simulink model "neurogrip_adaptive_mpc_closed_loop"  (R2026a)
settings: Solver=FixedStepDiscrete  StopTime=0.4  FixedStep=0.02
model workspace (MAT data in the model file):
  adaptiveMpc = mpc
  adaptiveMpc.Ts = 0.02
  adaptiveMpc.PredictionHorizon = 30
  adaptiveMpc.ControlHorizon = 30
  adaptiveMpc.Model.Plant = ss
  adaptiveMpc.Model.Plant.InputName_ = ["steering_angle_rad"; "d_kappa_rad_s"]
  adaptiveMpc.Model.Plant.InputGroup_.Manipulated = 1
  adaptiveMpc.Model.Plant.InputGroup_.Measured = 2
  adaptiveMpc.Model.Plant.OutputName_ = ["e_y_m"; "e_psi_rad"; "v_y_mps"; "yaw_rate_rps"]
  adaptiveMpc.Model.Plant.OutputGroup_.Measured = [1 2 3 4]
  adaptiveMpc.Model.Plant.IOSize_ = [4 2]
  adaptiveMpc.Model.Plant.Data_ = ltipack.ssdata
  adaptiveMpc.Model.Plant.Data_.a = [1  0.09  0.02  0; 0  1  0  0.02; 0  0  0.463654239616  -0.0414393740331; 0  0  0  0.457235651577]
  adaptiveMpc.Model.Plant.Data_.c = [1  0  0  0; 0  1  0  0; 0  0  1  0; 0  0  0  1]
  adaptiveMpc.Model.Plant.Data_.dx0 = [0; 0; 0; 0]
  adaptiveMpc.Model.Plant.Data_.x0 = [0; 0; 0; 0]
  adaptiveMpc.Model.Plant.Data_.b = [0  0; 0  -0.02; 1.14394485122  0; 1.59636573066  0]
  adaptiveMpc.Model.Plant.Data_.d = [0  0; 0  0; 0  0; 0  0]
  adaptiveMpc.Model.Plant.Data_.u0 = [0; 0]
  adaptiveMpc.Model.Plant.Data_.y0 = [0; 0; 0; 0]
  adaptiveMpc.Model.Plant.Data_.Delay.Input = [0; 0]
  adaptiveMpc.Model.Plant.Data_.Delay.Output = [0; 0; 0; 0]
  adaptiveMpc.Model.Plant.Data_.Delay.Internal = []
  adaptiveMpc.Model.Plant.Data_.Ts = 0.02
  adaptiveMpc.Model.Disturbance = []
  adaptiveMpc.Model.Noise = []
  adaptiveMpc.Model.Nominal.X = [0; 0; 0; 0]
  adaptiveMpc.Model.Nominal.DX = [0; 0; 0; 0]
  adaptiveMpc.Model.Nominal.U = [0; 0]
  adaptiveMpc.Model.Nominal.Y = [0; 0; 0; 0]
  adaptiveMpc.ManipulatedVariables.Min = -0.37
  adaptiveMpc.ManipulatedVariables.Max = 0.37
  adaptiveMpc.ManipulatedVariables.MinECR = 0
  adaptiveMpc.ManipulatedVariables.MaxECR = 0
  adaptiveMpc.ManipulatedVariables.RateMin = -0.05
  adaptiveMpc.ManipulatedVariables.RateMax = 0.05
  adaptiveMpc.ManipulatedVariables.RateMinECR = 0
  adaptiveMpc.ManipulatedVariables.RateMaxECR = 0
  adaptiveMpc.ManipulatedVariables.Target = 'nominal'
  adaptiveMpc.ManipulatedVariables.Name = 'steering_angle_rad'
  adaptiveMpc.ManipulatedVariables.Units = ''
  adaptiveMpc.ManipulatedVariables.ScaleFactor = 1
  adaptiveMpc.ManipulatedVariables.Type = 'continuous'
  adaptiveMpc.OutputVariables(1).Min = -1.5
  adaptiveMpc.OutputVariables(1).Max = 1.5
  adaptiveMpc.OutputVariables(1).MinECR = 1
  adaptiveMpc.OutputVariables(1).MaxECR = 1
  adaptiveMpc.OutputVariables(1).Name = 'e_y_m'
  adaptiveMpc.OutputVariables(1).Units = ''
  adaptiveMpc.OutputVariables(1).ScaleFactor = 1
  adaptiveMpc.OutputVariables(2).Min = -Inf
  adaptiveMpc.OutputVariables(2).Max = Inf
  adaptiveMpc.OutputVariables(2).MinECR = 1
  adaptiveMpc.OutputVariables(2).MaxECR = 1
  adaptiveMpc.OutputVariables(2).Name = 'e_psi_rad'
  adaptiveMpc.OutputVariables(2).Units = ''
  adaptiveMpc.OutputVariables(2).ScaleFactor = 1
  adaptiveMpc.OutputVariables(3).Min = -Inf
  adaptiveMpc.OutputVariables(3).Max = Inf
  adaptiveMpc.OutputVariables(3).MinECR = 1
  adaptiveMpc.OutputVariables(3).MaxECR = 1
  adaptiveMpc.OutputVariables(3).Name = 'v_y_mps'
  adaptiveMpc.OutputVariables(3).Units = ''
  adaptiveMpc.OutputVariables(3).ScaleFactor = 1
  adaptiveMpc.OutputVariables(4).Min = -Inf
  adaptiveMpc.OutputVariables(4).Max = Inf
  adaptiveMpc.OutputVariables(4).MinECR = 1
  adaptiveMpc.OutputVariables(4).MaxECR = 1
  adaptiveMpc.OutputVariables(4).Name = 'yaw_rate_rps'
  adaptiveMpc.OutputVariables(4).Units = ''
  adaptiveMpc.OutputVariables(4).ScaleFactor = 1
  adaptiveMpc.DisturbanceVariables.Name = 'd_kappa_rad_s'
  adaptiveMpc.DisturbanceVariables.Units = ''
  adaptiveMpc.DisturbanceVariables.ScaleFactor = 1
  adaptiveMpc.Weights.ManipulatedVariables = 20
  adaptiveMpc.Weights.ManipulatedVariablesRate = 5
  adaptiveMpc.Weights.OutputVariables = [40 60 5 10]
  adaptiveMpc.Weights.ECR = 100000
  adaptiveMpc.Optimizer.OptimizationType = 'QP'
  adaptiveMpc.Optimizer.Solver = 'active-set'
  adaptiveMpc.Optimizer.SolverOptions = mpc.solver.options.qp.ActiveSet
  adaptiveMpc.Optimizer.SolverOptions.SolverName = 'ActiveSet'
  adaptiveMpc.Optimizer.MinOutputECR = 0
  adaptiveMpc.Optimizer.UseSuboptimalSolution = 0
  adaptiveMpc.Optimizer.CustomSolver = 0
  adaptiveMpc.Optimizer.CustomSolverCodeGen = 0
  adaptiveMpc.History = [2026 10 3 11 47 55.738761]
  adaptiveMpc.MPCData = mpcdata
  adaptiveMpc.MPCData.IsDirty = 1
  adaptiveMpc.MPCData.Ts = 0.02
  adaptiveMpc.MPCData.p = 30
  adaptiveMpc.MPCData.m = 30
  adaptiveMpc.MPCData.UseActiveSetSolver = 1
  adaptiveMpc.MPCData.UseSuboptimalSolution = 0
  adaptiveMpc.MPCData.CustomSolver = 0
  adaptiveMpc.MPCData.CustomSolverCodeGen = 0
  adaptiveMpc.MPCData.IsCustomEstimation = 0
  adaptiveMpc.MPCData.Uscale = [1; 1]
  adaptiveMpc.MPCData.Yscale = [1; 1; 1; 1]
  adaptiveMpc.MPCData.mvindex = 1
  adaptiveMpc.MPCData.mdindex = 2
  adaptiveMpc.MPCData.myindex = [1; 2; 3; 4]
  adaptiveMpc.MPCData.ASOptions.MaxIterations = 120
  adaptiveMpc.MPCData.ASOptions.ConstraintTolerance = 1e-06
  adaptiveMpc.MPCData.ASOptions.UseWarmStart = 1
  adaptiveMpc.MPCData.IPOptions.MaxIterations = 50
  adaptiveMpc.MPCData.IPOptions.ConstraintTolerance = 1e-06
  adaptiveMpc.MPCData.IPOptions.OptimalityTolerance = 1e-06
  adaptiveMpc.MPCData.IPOptions.ComplementarityTolerance = 1e-08
  adaptiveMpc.MPCData.IPOptions.StepTolerance = 1e-08
  adaptiveMpc.MPCData.ADOptions.AbsoluteTolerance = 0.001
  adaptiveMpc.MPCData.ADOptions.RelativeTolerance = 0.001
  adaptiveMpc.MPCData.ADOptions.MaxIterations = 1000
  adaptiveMpc.MPCData.ADOptions.RelaxationParameter = 1.6
  adaptiveMpc.MPCData.ADOptions.PenaltyParameter = 0.1
  adaptiveMpc.MPCData.ADOptions.StepSize = 1e-06
  adaptiveMpc.MPCData.ADOptions.PrimalInfeasibilityTolerance = 0.0001
  adaptiveMpc.MPCData.ADOptions.DualInfeasibilityTolerance = 0.0001
  adaptiveMpc.MPCData.ADOptions.EnablePolish = 0
  adaptiveMpc.MPCData.ADOptions.PolishRegularization = 1e-06
  adaptiveMpc.MPCData.ADOptions.PolishTolerance = 1e-08
  adaptiveMpc.MPCData.ADOptions.PolishMaxIterations = 3
  adaptiveMpc.MPCData.MIQPOptions.MaxIterations = 1000
  adaptiveMpc.MPCData.MIQPOptions.ConstraintTolerance = 1e-06
  adaptiveMpc.MPCData.MIQPOptions.UseWarmStart = 0
  adaptiveMpc.MPCData.MIQPOptions.DiscreteConstraintTolerance = 1e-06
  adaptiveMpc.MPCData.MIQPOptions.RoundingAtRootNode = 1
  adaptiveMpc.MPCData.MIQPOptions.MaxPendingNodes = 1000
  adaptiveMpc.IsEmpty = 0
  adaptiveMpc.OldOVIntegrator = {[]; []; []; []}
  adaptiveMpc.Version = '26.1'
  onlineA = [1 0 0 0 0.09 1 0 0 0.02 0 0.463654239616 0 ... (496 elements, 4x4x31)]
  onlineB = reshape([0 0 1.14394485122 1.59636573066 0 -0.02 0 0 0 0 1.14394485122 1.59636573066 0 -0.02 0 0 0 0 1.14394485122 1.59636573066 0 -0.02 0 0 0 0 1.14394485122 1.59636573066 0 -0.02 0 0 0 0 1.14394485122 1.59636573066 0 -0.02 0 0 0 0 1.14394485122 1.59636573066 0 -0.02 0 0 0 0 1.14394485122 1.59636573066 0 -0.02 0 0 0 0 1.14394485122 1.59636573066 0 -0.02 0 0 0 0 1.14394485122 1.59636573066 0 -0.02 0 0 0 0 1.14394485122 1.59636573066 0 -0.02 0 0 0 0 1.14394485122 1.59636573066 0 -0.02 0 0 0 0 1.14394485122 1.59636573066 0 -0.02 0 0 0 0 1.14394485122 1.59636573066 0 -0.02 0 0 0 0 1.14394485122 1.59636573066 0 -0.02 0 0 0 0 1.14394485122 1.59636573066 0 -0.02 0 0 0 0 1.14394485122 1.59636573066 0 -0.02 0 0 0 0 1.14394485122 1.59636573066 0 -0.02 0 0 0 0 1.14394485122 1.59636573066 0 -0.02 0 0 0 0 1.14394485122 1.59636573066 0 -0.02 0 0 0 0 1.14394485122 1.59636573066 0 -0.02 0 0 0 0 1.14394485122 1.59636573066 0 -0.02 0 0 0 0 1.14394485122 1.59636573066 0 -0.02 0 0 0 0 1.14394485122 1.59636573066 0 -0.02 0 0 0 0 1.14394485122 1.59636573066 0 -0.02 0 0 0 0 1.14394485122 1.59636573066 0 -0.02 0 0 0 0 1.14394485122 1.59636573066 0 -0.02 0 0 0 0 1.14394485122 1.59636573066 0 -0.02 0 0 0 0 1.14394485122 1.59636573066 0 -0.02 0 0 0 0 1.14394485122 1.59636573066 0 -0.02 0 0 0 0 1.14394485122 1.59636573066 0 -0.02 0 0 0 0 1.14394485122 1.59636573066 0 -0.02 0 0], [4 2 31])
  onlineC = reshape([1 0 0 0 0 1 0 0 0 0 1 0 0 0 0 1 1 0 0 0 0 1 0 0 0 0 1 0 0 0 0 1 1 0 0 0 0 1 0 0 0 0 1 0 0 0 0 1 1 0 0 0 0 1 0 0 0 0 1 0 0 0 0 1 1 0 0 0 0 1 0 0 0 0 1 0 0 0 0 1 1 0 0 0 0 1 0 0 0 0 1 0 0 0 0 1 1 0 0 0 0 1 0 0 0 0 1 0 0 0 0 1 1 0 0 0 0 1 0 0 0 0 1 0 0 0 0 1 1 0 0 0 0 1 0 0 0 0 1 0 0 0 0 1 1 0 0 0 0 1 0 0 0 0 1 0 0 0 0 1 1 0 0 0 0 1 0 0 0 0 1 0 0 0 0 1 1 0 0 0 0 1 0 0 0 0 1 0 0 0 0 1 1 0 0 0 0 1 0 0 0 0 1 0 0 0 0 1 1 0 0 0 0 1 0 0 0 0 1 0 0 0 0 1 1 0 0 0 0 1 0 0 0 0 1 0 0 0 0 1 1 0 0 0 0 1 0 0 0 0 1 0 0 0 0 1 1 0 0 0 0 1 0 0 0 0 1 0 0 0 0 1 1 0 0 0 0 1 0 0 0 0 1 0 0 0 0 1 1 0 0 0 0 1 0 0 0 0 1 0 0 0 0 1 1 0 0 0 0 1 0 0 0 0 1 0 0 0 0 1 1 0 0 0 0 1 0 0 0 0 1 0 0 0 0 1 1 0 0 0 0 1 0 0 0 0 1 0 0 0 0 1 1 0 0 0 0 1 0 0 0 0 1 0 0 0 0 1 1 0 0 0 0 1 0 0 0 0 1 0 0 0 0 1 1 0 0 0 0 1 0 0 0 0 1 0 0 0 0 1 1 0 0 0 0 1 0 0 0 0 1 0 0 0 0 1 1 0 0 0 0 1 0 0 0 0 1 0 0 0 0 1 1 0 0 0 0 1 0 0 0 0 1 0 0 0 0 1 1 0 0 0 0 1 0 0 0 0 1 0 0 0 0 1 1 0 0 0 0 1 0 0 0 0 1 0 0 0 0 1 1 0 0 0 0 1 0 0 0 0 1 0 0 0 0 1], [4 4 31])
  onlineD = reshape([0 0 0 0 0 0 0 0 0 0 0 0 0 0 0 0 0 0 0 0 0 0 0 0 0 0 0 0 0 0 0 0 0 0 0 0 0 0 0 0 0 0 0 0 0 0 0 0 0 0 0 0 0 0 0 0 0 0 0 0 0 0 0 0 0 0 0 0 0 0 0 0 0 0 0 0 0 0 0 0 0 0 0 0 0 0 0 0 0 0 0 0 0 0 0 0 0 0 0 0 0 0 0 0 0 0 0 0 0 0 0 0 0 0 0 0 0 0 0 0 0 0 0 0 0 0 0 0 0 0 0 0 0 0 0 0 0 0 0 0 0 0 0 0 0 0 0 0 0 0 0 0 0 0 0 0 0 0 0 0 0 0 0 0 0 0 0 0 0 0 0 0 0 0 0 0 0 0 0 0 0 0 0 0 0 0 0 0 0 0 0 0 0 0 0 0 0 0 0 0 0 0 0 0 0 0 0 0 0 0 0 0 0 0 0 0 0 0 0 0 0 0 0 0 0 0 0 0 0 0 0 0 0 0 0 0 0 0 0 0 0 0 0 0 0 0 0 0], [4 2 31])
  onlineDX = reshape([0 0 0 0 0 0 0 0 0 0 0 0 0 0 0 0 0 0 0 0 0 0 0 0 0 0 0 0 0 0 0 0 0 0 0 0 0 0 0 0 0 0 0 0 0 0 0 0 0 0 0 0 0 0 0 0 0 0 0 0 0 0 0 0 0 0 0 0 0 0 0 0 0 0 0 0 0 0 0 0 0 0 0 0 0 0 0 0 0 0 0 0 0 0 0 0 0 0 0 0 0 0 0 0 0 0 0 0 0 0 0 0 0 0 0 0 0 0 0 0 0 0 0 0], [4 1 31])
  onlineU = reshape([0 0 0 0 0 0 0 0 0 0 0 0 0 0 0 0 0 0 0 0 0 0 0 0 0 0 0 0 0 0 0 0 0 0 0 0 0 0 0 0 0 0 0 0 0 0 0 0 0 0 0 0 0 0 0 0 0 0 0 0 0 0], [2 1 31])
  onlineX = reshape([0 0 0 0 0 0 0 0 0 0 0 0 0 0 0 0 0 0 0 0 0 0 0 0 0 0 0 0 0 0 0 0 0 0 0 0 0 0 0 0 0 0 0 0 0 0 0 0 0 0 0 0 0 0 0 0 0 0 0 0 0 0 0 0 0 0 0 0 0 0 0 0 0 0 0 0 0 0 0 0 0 0 0 0 0 0 0 0 0 0 0 0 0 0 0 0 0 0 0 0 0 0 0 0 0 0 0 0 0 0 0 0 0 0 0 0 0 0 0 0 0 0 0 0], [4 1 31])
  onlineY = reshape([0 0 0 0 0 0 0 0 0 0 0 0 0 0 0 0 0 0 0 0 0 0 0 0 0 0 0 0 0 0 0 0 0 0 0 0 0 0 0 0 0 0 0 0 0 0 0 0 0 0 0 0 0 0 0 0 0 0 0 0 0 0 0 0 0 0 0 0 0 0 0 0 0 0 0 0 0 0 0 0 0 0 0 0 0 0 0 0 0 0 0 0 0 0 0 0 0 0 0 0 0 0 0 0 0 0 0 0 0 0 0 0 0 0 0 0 0 0 0 0 0 0 0 0], [4 1 31])
libraries: mpclib x1
settings Model: Creator=pavel  LastModifiedBy=pavel

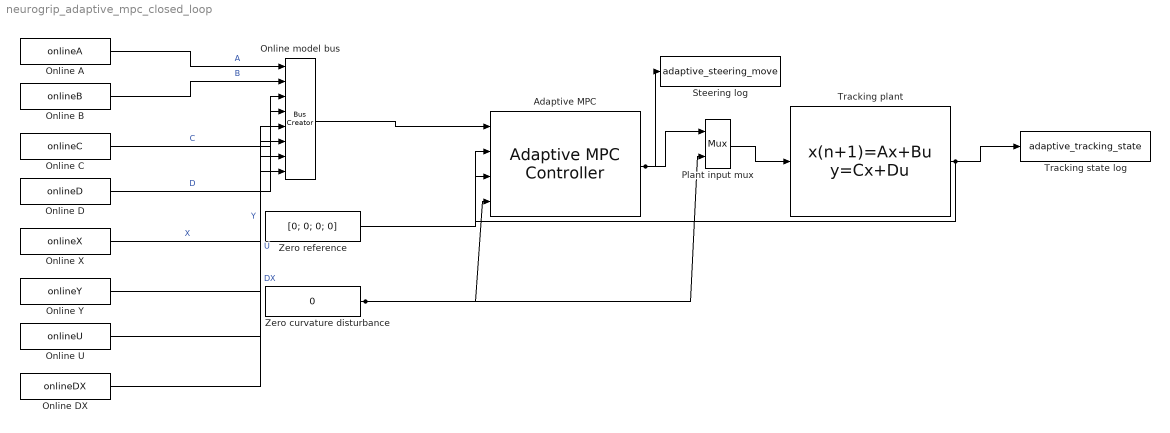
== system neurogrip_adaptive_mpc_closed_loop ==
  Adaptive MPC : mpclib/Adaptive MPC Controller  SCDEnableBlockLinearizationSpecification=on  mpcobj=adaptiveMpc  enable_value=0  updateMPCinCallerWorkspace=on  md_inport=on  mv_inport=off  uref_inport=off  return_cost=off  return_mvseq=off  return_qpstatus=off  return_xseq=off  return_state=off  return_ovseq=off  state_inport=off  isltv_plant=on  umin_inport=off  umax_inport=off  ymin_inport=off  ymax_inport=off  cc_inport=off  ywt_inport=off  uwt_inport=off  duwt_inport=off  rhoeps_inport=off  pm_inport=off  MaximumP=10  HorizonChoice=FixedHorizon  BlockDataType=double  SampleTimeInherited=off  switch_inport=off
  Online A : Constant  Value=onlineA
  Online B : Constant  Value=onlineB
  Online C : Constant  Value=onlineC
  Online D : Constant  Value=onlineD
  Online DX : Constant  Value=onlineDX
  Online U : Constant  Value=onlineU
  Online X : Constant  Value=onlineX
  Online Y : Constant  Value=onlineY
  Online model bus : BusCreator  Inputs=8
  Plant input mux : Mux  Inputs=2
  Steering log : ToWorkspace  VariableName=adaptive_steering_move  SaveFormat=Structure With Time  SampleTime=-1
  Tracking plant : DiscreteStateSpace  A=[1 0.089999999999999997 0.02 0;0 1 0 0.02;0 0 0.46365423961556773 -0.041439374033090781;0 0 0 0.4572356515766039]  B=[0 0;0 -0.02;1.1439448512165971 0;1.5963657306570473 0]  C=eye(4)  D=zeros(4, 2)  InitialCondition=[0.20; 0.05; 0.00; 0.00]  SampleTime=0.02
  Tracking state log : ToWorkspace  VariableName=adaptive_tracking_state  SaveFormat=Structure With Time  SampleTime=-1
  Zero curvature disturbance : Constant  Value=0
  Zero reference : Constant  Value=[0; 0; 0; 0]
  wires:
  Online A/1 -> Online model bus/1  "A"
  Online B/1 -> Online model bus/2  "B"
  Online C/1 -> Online model bus/3  "C"
  Online D/1 -> Online model bus/4  "D"
  Online X/1 -> Online model bus/5  "X"
  Online Y/1 -> Online model bus/6  "Y"
  Online U/1 -> Online model bus/7  "U"
  Online DX/1 -> Online model bus/8  "DX"
  Online model bus/1 -> Adaptive MPC/1
  Tracking plant/1 -> Adaptive MPC/2, Tracking state log/1
  Zero reference/1 -> Adaptive MPC/3
  Zero curvature disturbance/1 -> Adaptive MPC/4, Plant input mux/2
  Adaptive MPC/1 -> Plant input mux/1, Steering log/1
  Plant input mux/1 -> Tracking plant/1
